simulink model "controllo_model_following"  (R2021a)
settings: Solver=VariableStepAuto  StartTime=0.0  StopTime=tsim  RelTol=1e-3
values from neighbouring files (symbols this model uses):
  A_tilde = -1    [main.m]
  Arc = 0    [main.m]
  b = 20    [main.m]
  B_tilde = 1    [main.m]
  Brc = 0    [main.m]
  c = 718    [main.m]
  C_tilde = 1    [main.m]
  Crc = 1    [main.m]
  D_tilde = 0    [main.m]
  Drc = 0    [main.m]
  F_aug_acc_fb_infinito = F_aug_acc_fb(1,:)    [main.m]
  F_aug_mf_fb_infinito = F_aug_mf_fb(1,:)    [main.m]
  f_w = 0    [main.m]
  g = 9.81    [main.m]
  k = 2.5    [main.m]
  m = 500    [main.m]
  p_a = 1.184    [main.m]
  Tc = 0.01    [main.m]
  theta_a = 298    [main.m]
  u_eq = k*(theta - theta_a)    (= 199.411134904)    [main.m]
  V = 2000    [main.m]
  x_0 = [550;0;150]    [main.m]
  x_eq = [600;0;theta]    [main.m]
undefined symbols (not defined in the file or in its folder): Cd, nmf
settings Model: Creator=Randy  LastModifiedBy=Randy

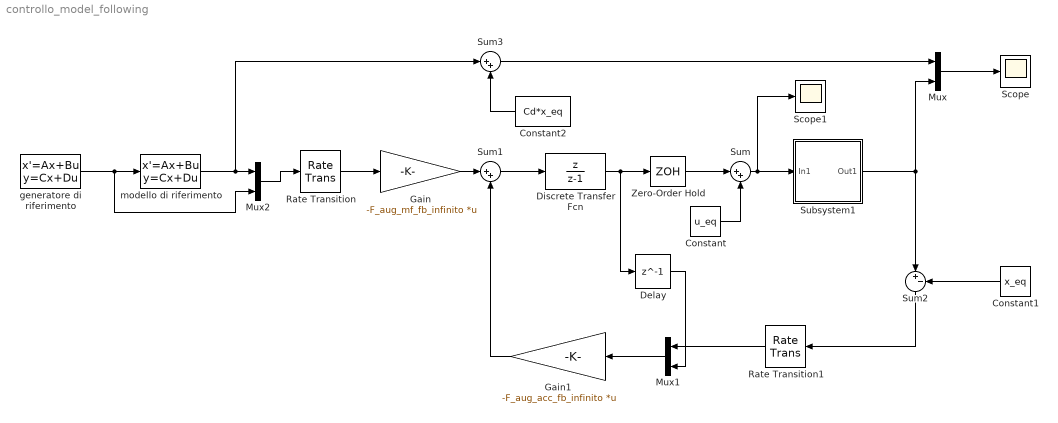
== system controllo_model_following ==
  Constant : Constant  Value=u_eq
  Constant1 : Constant  Value=x_eq  VectorParams1D=off
  Constant2 : Constant  Value=Cd*x_eq
  Delay : Delay  DelayLength=1  SampleTime=Tc
  Discrete Transfer Fcn : DiscreteTransferFcn  Numerator=[1 0]  Denominator=[1 -1]  SampleTime=Tc
  Gain : Gain  Gain=-F_aug_mf_fb_infinito  Multiplication=Matrix(K*u)
  Gain1 : Gain  Gain=-F_aug_acc_fb_infinito  Multiplication=Matrix(K*u)
  Mux : Mux  Inputs=2
  Mux1 : Mux  Inputs=2
  Mux2 : Mux  Inputs=2
  Rate Transition : RateTransition  OutPortSampleTime=Tc
  Rate Transition1 : RateTransition  OutPortSampleTime=Tc
  Scope : Scope
  Scope1 : Scope
  Subsystem1 : Subsystem
  Sum : Sum  Inputs=|++
  Sum1 : Sum  Inputs=|++
  Sum2 : Sum  Inputs=|+-
  Sum3 : Sum  Inputs=|++
  Zero-Order Hold : ZeroOrderHold  SampleTime=Tc
  generatore di riferimento : StateSpace  A=Arc  B=Brc  C=Crc  D=Drc  InitialCondition=600
  modello di riferimento : StateSpace  A=A_tilde  B=B_tilde  C=[C_tilde; eye(nmf)]  D=[D_tilde;0]  InitialCondition=0
  wires:
  Rate Transition1/1 -> Mux1/1
  Constant1/1 -> Sum2/2
  Sum2/1 -> Rate Transition1/1
  Sum3/1 -> Mux/1
  Constant/1 -> Sum/2
  Delay/1 -> Mux1/2
  Mux1/1 -> Gain1/1
  Constant2/1 -> Sum3/2
  modello di riferimento/1 -> Sum3/1, Mux2/1
  Gain/1 -> Sum1/1
  Mux/1 -> Scope/1
  Gain1/1 -> Sum1/2
  Sum1/1 -> Discrete Transfer Fcn/1
  Zero-Order Hold/1 -> Sum/1
  Discrete Transfer Fcn/1 -> Delay/1, Zero-Order Hold/1
  Rate Transition/1 -> Gain/1
  Sum/1 -> Scope1/1, Subsystem1/1(In1)
  Subsystem1/1(Out1) -> Mux/2, Sum2/1
  Mux2/1 -> Rate Transition/1
  generatore di riferimento/1 -> modello di riferimento/1, Mux2/2

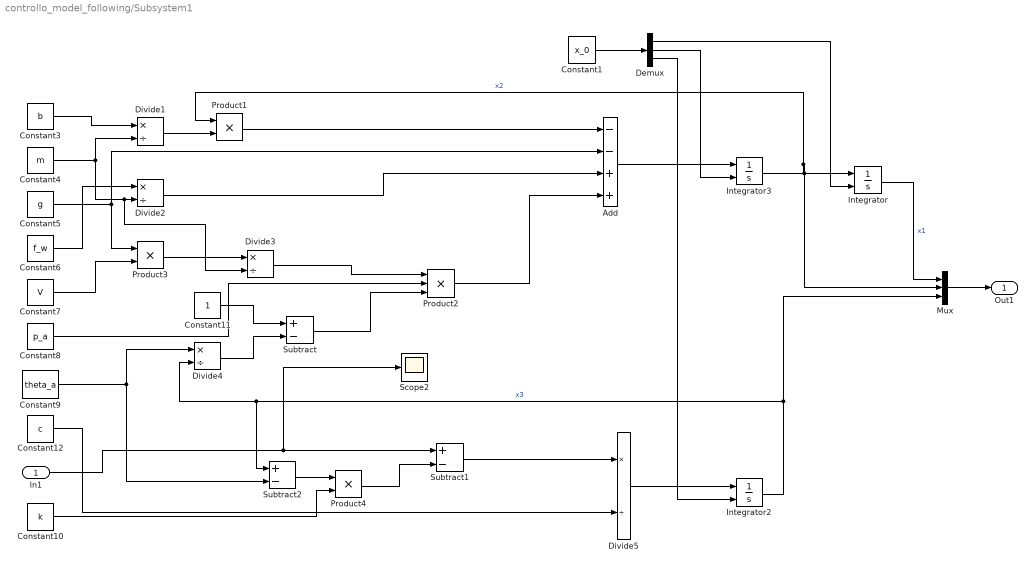
== system controllo_model_following/Subsystem1 ==
  In1 : Inport
  Add : Sum  Inputs=--++
  Constant1 : Constant  Value=x_0
  Constant10 : Constant  Value=k
  Constant11 : Constant
  Constant12 : Constant  Value=c
  Constant3 : Constant  Value=b
  Constant4 : Constant  Value=m
  Constant5 : Constant  Value=g
  Constant6 : Constant  Value=f_w
  Constant7 : Constant  Value=V
  Constant8 : Constant  Value=p_a
  Constant9 : Constant  Value=theta_a
  Demux : Demux  Outputs=3
  Divide{1..5} (5 alike) : Product  Inputs=*/
  Integrator : Integrator  InitialConditionSource=external  InitialCondition=680
  Integrator2 : Integrator  InitialConditionSource=external  InitialCondition=400
  Integrator3 : Integrator  InitialConditionSource=external
  Mux : Mux  Inputs=3
  Product1 : Product
  Product2 : Product  Inputs=3
  Product3 : Product
  Product4 : Product
  Scope2 : Scope
  Subtract : Sum  Inputs=+-
  Subtract1 : Sum  Inputs=+-
  Subtract2 : Sum  Inputs=+-
  Out1 : Outport
  wires:
  Subtract/1 -> Product2/3
  In1/1 -> Scope2/1, Subtract1/1
  Constant9/1 -> Subtract2/2, Divide4/1
  Constant5/1 -> Product3/1, Add/2
  Divide4/1 -> Subtract/2
  Constant10/1 -> Product4/2
  Constant7/1 -> Product3/2
  Product2/1 -> Add/4
  Subtract2/1 -> Product4/1
  Divide1/1 -> Product1/2
  Constant3/1 -> Divide1/1
  Product4/1 -> Subtract1/2
  Constant11/1 -> Subtract/1
  Integrator3/1 -> Mux/2, Integrator/1, Product1/1  "x2"
  Divide2/1 -> Add/3
  Integrator/1 -> Mux/1  "x1"
  Constant4/1 -> Divide3/2, Divide2/2, Divide1/2
  Product3/1 -> Divide3/1
  Product1/1 -> Add/1
  Divide3/1 -> Product2/1
  Mux/1 -> Out1/1
  Add/1 -> Integrator3/1
  Constant8/1 -> Product2/2
  Divide5/1 -> Integrator2/1
  Constant12/1 -> Divide5/2
  Constant6/1 -> Divide2/1
  Subtract1/1 -> Divide5/1
  Integrator2/1 -> Mux/3, Subtract2/1, Divide4/2  "x3"
  Constant1/1 -> Demux/1
  Demux/1 -> Integrator/2
  Demux/2 -> Integrator3/2
  Demux/3 -> Integrator2/2
